simulink model "FLWSim_PoincareMap"  (R2017b)
settings: Solver=ode45  StartTime=0.0  StopTime=30  MaxStep=0.001  RelTol=1e-3
InitFcn:
  | SimInit
  | PolyRegressionFilterInit
  | CustomInit
undefined symbols (not defined in the file): dq, IC, q, sample_time
libraries: commchan3 x8, simulink x2, dspsigattribs x2
settings Model: Creator=81068  LastModifiedBy=81068
settings SFSimCC: SimUserSources=|
  | CoriolisTerm_src.c
  | GravityVector_src.c
  | InertiaMatrix_src.c
  | 
  | AMBody_LeftShin_src.c
  | AMBody_LeftThigh_src.c
  | AMBody_RightShin_src.c
  | AMBody_RightThigh_src.c
  | AMBody_Torso_src.c
  | AMworld_about_pA_src.c
  | AMWorld_LeftShin_src.c
  | AMWorld_LeftThigh_src.c
  | AMWorld_RightShin_src.c
  | AMWorld_RightThigh_src.c
  | AMWorld_Torso_src.c
  | dJb_Head_src.c
  | dJb_LeftHip_src.c
  | dJb_LeftKnee_src.c
  | dJb_LeftShin_src.c
  | dJb_LeftThigh_src.c
  | dJb_LeftToe_src.c
  | dJb_RightHip_src.c
  | dJb_RightKnee_src.c
  | dJb_RightShin_src.c
  | dJb_RightThigh_src.c
  | dJb_RightToe_src.c
  | dJb_Torso_src.c
  | dJp_COM_src.c
  | dJp_Head_src.c
  | dJp_LeftHip_src.c
  | dJp_LeftKnee_src.c
  | dJp_LeftShin_src.c
  | dJp_LeftThigh_src.c
  | dJp_LeftToe_src.c
  | dJp_RightHip_src.c
  | dJp_RightKnee_src.c
  | dJp_RightShin_src.c
  | dJp_RightThigh_src.c
  | dJp_RightToe_src.c
  | dJp_Torso_src.c
  | dJs_Head_src.c
  | dJs_LeftHip_src.c
  | dJs_LeftKnee_src.c
  | dJs_LeftShin_src.c
  | dJs_LeftThigh_src.c
  | dJs_LeftToe_src.c
  | dJs_RightHip_src.c
  | dJs_RightKnee_src.c
  | dJs_RightShin_src.c
  | dJs_RightThigh_src.c
  | dJs_RightToe_src.c
  | dJs_Torso_src.c
  | dR_Head_src.c
  | dR_LeftHip_src.c
  | dR_LeftKnee_src.c
  | dR_LeftShin_src.c
  | dR_LeftThigh_src.c
  | dR_LeftToe_src.c
  | dR_RightHip_src.c
  | dR_RightKnee_src.c
  | dR_RightShin_src.c
  | dR_RightThigh_src.c
  | dR_RightToe_src.c
  | dR_Torso_src.c
  | dT_Head_src.c
  | dT_LeftHip_src.c
  | dT_LeftKnee_src.c
  | dT_LeftShin_src.c
  | dT_LeftThigh_src.c
  | dT_LeftToe_src.c
  | dT_RightHip_src.c
  | dT_RightKnee_src.c
  | dT_RightShin_src.c
  | dT_RightThigh_src.c
  | dT_RightToe_src.c
  | dT_Torso_src.c
  | Inertia_LeftShin_src.c
  | Inertia_LeftThigh_src.c
  | Inertia_RightShin_src.c
  | Inertia_RightThigh_src.c
  | Inertia_Torso_src.c
  | Jb_Head_src.c
  | Jb_LeftHip_src.c
  | Jb_LeftKnee_src.c
  | Jb_LeftShin_src.c
  | Jb_LeftThigh_src.c
  | Jb_LeftToe_src.c
  | Jb_RightHip_src.c
  | Jb_RightKnee_src.c
  | Jb_RightShin_src.c
  | Jb_RightThigh_src.c
  | Jb_RightToe_src.c
  | Jb_Torso_src.c
  | Jdq_AMBody_LeftShin_src.c
  | Jdq_AMBody_LeftThigh_src.c
  | Jdq_AMBody_RightShin_src.c
  | Jdq_AMBody_RightThigh_src.c
  | Jdq_AMBody_Torso_src.c
  | Jdq_AMworld_about_pA_src.c
  | Jdq_AMWorld_LeftShin_src.c
  | Jdq_AMWorld_LeftThigh_src.c
  | Jdq_AMWorld_RightShin_src.c
  | Jdq_AMWorld_RightThigh_src.c
  | Jdq_AMWorld_Torso_src.c
  | Jp_COM_src.c
  | Jp_Head_src.c
  | Jp_LeftHip_src.c
  | Jp_LeftKnee_src.c
  | Jp_LeftShin_src.c
  | Jp_LeftThigh_src.c
  | Jp_LeftToe_src.c
  | Jp_RightHip_src.c
  | Jp_RightKnee_src.c
  | Jp_RightShin_src.c
  | Jp_RightThigh_src.c
  | Jp_RightToe_src.c
  | Jp_Torso_src.c
  | Jq_AMBody_LeftShin_src.c
  | Jq_AMBody_LeftThigh_src.c
  | Jq_AMBody_RightShin_src.c
  | Jq_AMBody_RightThigh_src.c
  | Jq_AMBody_Torso_src.c
  | Jq_AMworld_about_pA_src.c
  | Jq_AMWorld_LeftShin_src.c
  | Jq_AMWorld_LeftThigh_src.c
  | Jq_AMWorld_RightShin_src.c
  | Jq_AMWorld_RightThigh_src.c
  | Jq_AMWorld_Torso_src.c
  | Js_Head_src.c
  | Js_LeftHip_src.c
  | Js_LeftKnee_src.c
  | Js_LeftShin_src.c
  | Js_LeftThigh_src.c
  | Js_LeftToe_src.c
  | Js_RightHip_src.c
  | Js_RightKnee_src.c
  | Js_RightShin_src.c
  | Js_RightThigh_src.c
  | Js_RightToe_src.c
  | Js_Torso_src.c
  | p_COM_src.c
  | p_Head_src.c
  | p_LeftHip_src.c
  | p_LeftKnee_src.c
  | p_LeftShin_src.c
  | p_LeftThigh_src.c
  | p_LeftToe_src.c
  | p_RightHip_src.c
  | p_RightKnee_src.c
  | p_RightShin_src.c
  | p_RightThigh_src.c
  | p_RightToe_src.c
  | p_Torso_src.c
  | R_Head_src.c
  | R_LeftHip_src.c
  | R_LeftKnee_src.c
  | R_LeftShin_src.c
  | R_LeftThigh_src.c
  | R_LeftToe_src.c
  | R_RightHip_src.c
  | R_RightKnee_src.c
  | R_RightShin_src.c
  | R_RightThigh_src.c
  | R_RightToe_src.c
  | R_Torso_src.c
  | T_Head_src.c
  | T_LeftHip_src.c
  | T_LeftKnee_src.c
  | T_LeftShin_src.c
  | T_LeftThigh_src.c
  | T_LeftToe_src.c
  | T_RightHip_src.c
  | T_RightKnee_src.c
  | T_RightShin_src.c
  | T_RightThigh_src.c
  | T_RightToe_src.c
  | T_Torso_src.c
settings SFSimCC: SimUserIncludeDirs=|
  | .\dyn\src
  | .\kin\src
settings RTWCC: RTWUseSimCustomCode=on
settings RTWCC: CustomInclude=|
  | .\dyn\src
  | .\kin\src
settings RTWCC: CustomSource=|
  | CoriolisTerm_src.c
  | GravityVector_src.c
  | InertiaMatrix_src.c
  | 
  | AMBody_LeftShin_src.c
  | AMBody_LeftThigh_src.c
  | AMBody_RightShin_src.c
  | AMBody_RightThigh_src.c
  | AMBody_Torso_src.c
  | AMworld_about_pA_src.c
  | AMWorld_LeftShin_src.c
  | AMWorld_LeftThigh_src.c
  | AMWorld_RightShin_src.c
  | AMWorld_RightThigh_src.c
  | AMWorld_Torso_src.c
  | dJb_Head_src.c
  | dJb_LeftHip_src.c
  | dJb_LeftKnee_src.c
  | dJb_LeftShin_src.c
  | dJb_LeftThigh_src.c
  | dJb_LeftToe_src.c
  | dJb_RightHip_src.c
  | dJb_RightKnee_src.c
  | dJb_RightShin_src.c
  | dJb_RightThigh_src.c
  | dJb_RightToe_src.c
  | dJb_Torso_src.c
  | dJp_COM_src.c
  | dJp_Head_src.c
  | dJp_LeftHip_src.c
  | dJp_LeftKnee_src.c
  | dJp_LeftShin_src.c
  | dJp_LeftThigh_src.c
  | dJp_LeftToe_src.c
  | dJp_RightHip_src.c
  | dJp_RightKnee_src.c
  | dJp_RightShin_src.c
  | dJp_RightThigh_src.c
  | dJp_RightToe_src.c
  | dJp_Torso_src.c
  | dJs_Head_src.c
  | dJs_LeftHip_src.c
  | dJs_LeftKnee_src.c
  | dJs_LeftShin_src.c
  | dJs_LeftThigh_src.c
  | dJs_LeftToe_src.c
  | dJs_RightHip_src.c
  | dJs_RightKnee_src.c
  | dJs_RightShin_src.c
  | dJs_RightThigh_src.c
  | dJs_RightToe_src.c
  | dJs_Torso_src.c
  | dR_Head_src.c
  | dR_LeftHip_src.c
  | dR_LeftKnee_src.c
  | dR_LeftShin_src.c
  | dR_LeftThigh_src.c
  | dR_LeftToe_src.c
  | dR_RightHip_src.c
  | dR_RightKnee_src.c
  | dR_RightShin_src.c
  | dR_RightThigh_src.c
  | dR_RightToe_src.c
  | dR_Torso_src.c
  | dT_Head_src.c
  | dT_LeftHip_src.c
  | dT_LeftKnee_src.c
  | dT_LeftShin_src.c
  | dT_LeftThigh_src.c
  | dT_LeftToe_src.c
  | dT_RightHip_src.c
  | dT_RightKnee_src.c
  | dT_RightShin_src.c
  | dT_RightThigh_src.c
  | dT_RightToe_src.c
  | dT_Torso_src.c
  | Inertia_LeftShin_src.c
  | Inertia_LeftThigh_src.c
  | Inertia_RightShin_src.c
  | Inertia_RightThigh_src.c
  | Inertia_Torso_src.c
  | Jb_Head_src.c
  | Jb_LeftHip_src.c
  | Jb_LeftKnee_src.c
  | Jb_LeftShin_src.c
  | Jb_LeftThigh_src.c
  | Jb_LeftToe_src.c
  | Jb_RightHip_src.c
  | Jb_RightKnee_src.c
  | Jb_RightShin_src.c
  | Jb_RightThigh_src.c
  | Jb_RightToe_src.c
  | Jb_Torso_src.c
  | Jdq_AMBody_LeftShin_src.c
  | Jdq_AMBody_LeftThigh_src.c
  | Jdq_AMBody_RightShin_src.c
  | Jdq_AMBody_RightThigh_src.c
  | Jdq_AMBody_Torso_src.c
  | Jdq_AMworld_about_pA_src.c
  | Jdq_AMWorld_LeftShin_src.c
  | Jdq_AMWorld_LeftThigh_src.c
  | Jdq_AMWorld_RightShin_src.c
  | Jdq_AMWorld_RightThigh_src.c
  | Jdq_AMWorld_Torso_src.c
  | Jp_COM_src.c
  | Jp_Head_src.c
  | Jp_LeftHip_src.c
  | Jp_LeftKnee_src.c
  | Jp_LeftShin_src.c
  | Jp_LeftThigh_src.c
  | Jp_LeftToe_src.c
  | Jp_RightHip_src.c
  | Jp_RightKnee_src.c
  | Jp_RightShin_src.c
  | Jp_RightThigh_src.c
  | Jp_RightToe_src.c
  | Jp_Torso_src.c
  | Jq_AMBody_LeftShin_src.c
  | Jq_AMBody_LeftThigh_src.c
  | Jq_AMBody_RightShin_src.c
  | Jq_AMBody_RightThigh_src.c
  | Jq_AMBody_Torso_src.c
  | Jq_AMworld_about_pA_src.c
  | Jq_AMWorld_LeftShin_src.c
  | Jq_AMWorld_LeftThigh_src.c
  | Jq_AMWorld_RightShin_src.c
  | Jq_AMWorld_RightThigh_src.c
  | Jq_AMWorld_Torso_src.c
  | Js_Head_src.c
  | Js_LeftHip_src.c
  | Js_LeftKnee_src.c
  | Js_LeftShin_src.c
  | Js_LeftThigh_src.c
  | Js_LeftToe_src.c
  | Js_RightHip_src.c
  | Js_RightKnee_src.c
  | Js_RightShin_src.c
  | Js_RightThigh_src.c
  | Js_RightToe_src.c
  | Js_Torso_src.c
  | p_COM_src.c
  | p_Head_src.c
  | p_LeftHip_src.c
  | p_LeftKnee_src.c
  | p_LeftShin_src.c
  | p_LeftThigh_src.c
  | p_LeftToe_src.c
  | p_RightHip_src.c
  | p_RightKnee_src.c
  | p_RightShin_src.c
  | p_RightThigh_src.c
  | p_RightToe_src.c
  | p_Torso_src.c
  | R_Head_src.c
  | R_LeftHip_src.c
  | R_LeftKnee_src.c
  | R_LeftShin_src.c
  | R_LeftThigh_src.c
  | R_LeftToe_src.c
  | R_RightHip_src.c
  | R_RightKnee_src.c
  | R_RightShin_src.c
  | R_RightThigh_src.c
  | R_RightToe_src.c
  | R_Torso_src.c
  | T_Head_src.c
  | T_LeftHip_src.c
  | T_LeftKnee_src.c
  | T_LeftShin_src.c
  | T_LeftThigh_src.c
  | T_LeftToe_src.c
  | T_RightHip_src.c
  | T_RightKnee_src.c
  | T_RightShin_src.c
  | T_RightThigh_src.c
  | T_RightToe_src.c
  | T_Torso_src.c
settings CodeAppCC: StateflowObjectComments=on

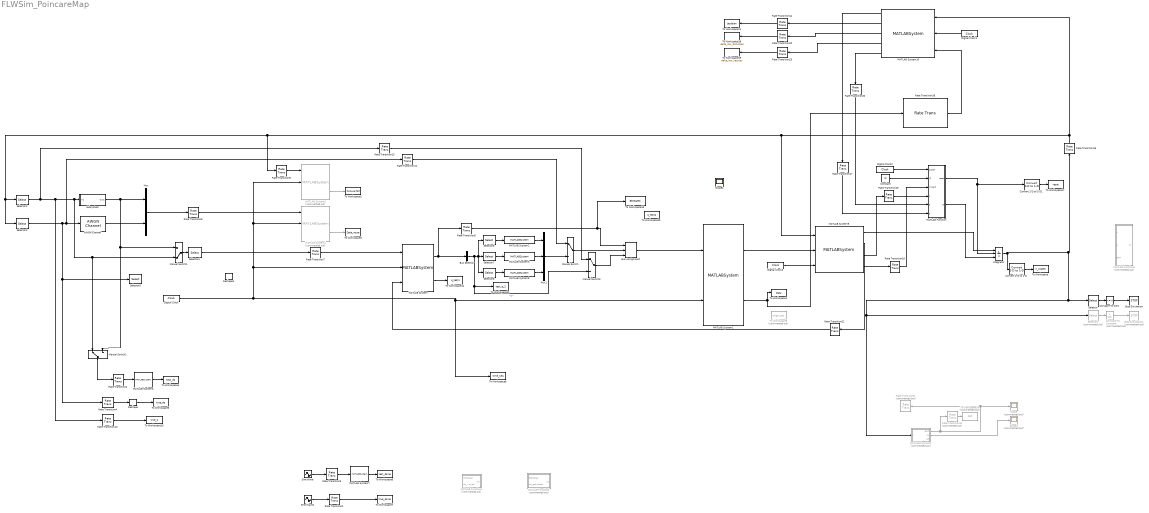
== system FLWSim_PoincareMap ==
  AWGN Channel : commchan3/AWGN Channel  InputProcessing=Columns as channels (frame based)  seed=4  noiseMode=Variance from mask  EbNodB=10  EsNodB=10  SNRdB=10  bitsPerSym=1  Ps=1  Tsym=1  variance=cov_dq_estimated
  Bus Assignment : BusAssignment  AssignedSignals=dq,q
  Bus Selector : BusSelector  OutputSignals=q
  Compare To Constant : simulink/Logic and Bit Operations/Compare To Constant  Commented=on  relop=>  const=100  OutDataTypeStr=boolean
  Compare To Zero : simulink/Logic and Bit Operations/Compare To Zero  relop=<=  OutDataTypeStr=boolean
  Constant : Constant  Value=IC
  Convert 2-D to 1-D : dspsigattribs/Convert 2-D to 1-D
      settings: SourceProductName=DSP System Toolbox  SourceProductBaseCode=DS
  Convert 2-D to 1-D1 : dspsigattribs/Convert 2-D to 1-D
      settings: SourceProductName=DSP System Toolbox  SourceProductBaseCode=DS
  Digital Clock{,1..3} (4 alike) : DigitalClock  SampleTime=sample_time
  Integrator : Integrator  ExternalReset=level hold  InitialConditionSource=external  InitialCondition=IC
  MATLAB Function : MATLAB Function  TreatAsAtomicUnit=on
  MATLAB Function1 : MATLAB Function  Commented=on  TreatAsAtomicUnit=on
  MATLAB Function4 : MATLAB Function  Commented=on  TreatAsAtomicUnit=on
  MATLAB Function5 : MATLAB Function  Commented=on  TreatAsAtomicUnit=on
  MATLAB Function6 : MATLAB Function  Commented=on  TreatAsAtomicUnit=on
  MATLAB System : MATLABSystem  System=StateEstimator_1  T=0.3  SimulateUsing=Interpreted execution
      mask Type: StateEstimator_1
      mask Display:
      | disp('StateEstimator_1');
      | port_label('input',1,'q_measured');
      | port_label('input',2,'t');
      | port_label('input',3,'GRF');
      | port_label('output',1,'EstStates');
      | port_label('output',2,'q');
  MATLAB System1 : MATLABSystem  System=FLW_Controller_Poincare  cov_q_measured=cov_q_measured  cov_dq_estimated=cov_dq_estimated  T_sample=sample_time  T=0.3  RegressFilterHistoryLength=history_length  fp_ratio=fp_ratio  SimulateUsing=Code generation
      mask Type: FLW_Controller_Poincare
      mask Display:
      | disp('FLW_Controller_Poincare');
      | port_label('input',1,'EstStates');
      | port_label('input',2,'t');
      | port_label('output',1,'u');
      | port_label('output',2,'Data');
  MATLAB System10 : MATLABSystem  System=Poincare_test  poincare_delta=poincare_delta  SimulateUsing=Code generation
      mask Type: Poincare_test
      mask Display:
      | disp('Poincare_test');
      | port_label('input',1,'x');
      | port_label('input',2,'t_total');
      | port_label('input',3,'Data');
      | port_label('output',1,'x_out');
      | port_label('output',2,'Jacobian');
      | port_label('output',3,'delta_low_disturbed');
      | port_label('output',4,'delta_low_recover');
      | port_label('output',5,'add_disturb');
  MATLAB System2 : MATLABSystem  System=PolyRegressionFilter  sample_time=sample_time  history_length=history_length  dop=dop  signal_dim=2  delay=RegressionDelay  SimulateUsing=Code generation
      mask Type: PolyRegressionFilter
      mask Display:
      | disp('PolyRegressionFilter');
      | port_label('input',1,'q');
      | port_label('output',1,'dq');
  MATLAB System3 : MATLABSystem  System=PolyRegressionFilter  sample_time=sample_time  history_length=history_length  dop=dop  signal_dim=1  delay=RegressionDelay  SimulateUsing=Code generation
      mask Type: PolyRegressionFilter
      mask Display:
      | disp('PolyRegressionFilter');
      | port_label('input',1,'q');
      | port_label('output',1,'dq');
  MATLAB System4 : MATLABSystem  Commented=on  System=FLW_Controller_3  cov_q=cov_q_measured  cov_dq=cov_dq_estimated  T_sample=sample_time  SimulateUsing=Code generation
      mask Type: FLW_Controller_3
      mask Display:
      | disp('FLW_Controller_3');
      | port_label('input',1,'x');
      | port_label('input',2,'t');
      | port_label('input',3,'GRF');
      | port_label('output',1,'u');
      | port_label('output',2,'Data');
  MATLAB System5 : MATLABSystem  Commented=on  System=FLW_Controller_3  cov_q=cov_q_measured  cov_dq=cov_dq_estimated  T_sample=sample_time  SimulateUsing=Code generation
      mask Type: FLW_Controller_3
      mask Display:
      | disp('FLW_Controller_3');
      | port_label('input',1,'x');
      | port_label('input',2,'t');
      | port_label('input',3,'GRF');
      | port_label('output',1,'u');
      | port_label('output',2,'Data');
  MATLAB System6 : MATLABSystem  System=PolyRegressionFilter  sample_time=sample_time  history_length=history_length  dop=dop  signal_dim=7  delay=RegressionDelay  SimulateUsing=Code generation
      mask Type: PolyRegressionFilter
      mask Display:
      | disp('PolyRegressionFilter');
      | port_label('input',1,'q');
      | port_label('output',1,'dq');
  MATLAB System7 : MATLABSystem  System=PolyRegressionFilter  sample_time=sample_time  history_length=history_length  dop=dop  signal_dim=1  delay=20  SimulateUsing=Code generation
      mask Type: PolyRegressionFilter
      mask Display:
      | disp('PolyRegressionFilter');
      | port_label('input',1,'q');
      | port_label('output',1,'dq');
  MATLAB System8 : MATLABSystem  System=PolyRegressionFilter  sample_time=sample_time  history_length=history_length  dop=dop  signal_dim=4  delay=RegressionDelay  SimulateUsing=Code generation
      mask Type: PolyRegressionFilter
      mask Display:
      | disp('PolyRegressionFilter');
      | port_label('input',1,'q');
      | port_label('output',1,'dq');
  MATLAB System9 : MATLABSystem  System=EOM_Rigid_Ground  IC=IC  SimulateUsing=Code generation
      mask Type: EOM_Rigid_Ground
      mask Display:
      | disp('EOM_Rigid_Ground');
      | port_label('input',1,'x');
      | port_label('input',2,'u');
      | port_label('input',3,'t_total');
      | port_label('output',1,'dx');
      | port_label('output',2,'GRF');
      | port_label('output',3,'x_reset');
      | port_label('output',4,'impact');
  Manual Switch : ManualSwitch
  Manual Switch1 : ManualSwitch  CurrentSetting=0
  Manual Switch2 : ManualSwitch
  Manual Switch3 : ManualSwitch
  Mux : Mux  Inputs=2
  Mux1 : Mux  Inputs=3
  Rate Transition{1..8,10..11,13..15,22..23} (15 alike) : RateTransition  OutPortSampleTime=sample_time
  Rate Transition12 : RateTransition  Commented=on  OutPortSampleTime=sample_time
  Rate Transition{16..21} (6 alike) : RateTransition  OutPortSampleTimeOpt=Inherit
  Rate Transition9 : RateTransition  Commented=on  OutPortSampleTime=sample_time
  Reshape : Reshape  OutputDimensionality=Column vector (2-D)
  Reshape1 : Reshape  OutputDimensionality=Column vector (2-D)
  Scope : Scope  Commented=on
  Scope1 : Scope  Commented=on
  Scope2 : Scope
  Selector : Selector  InputPortWidth=14  IndexOptions=Index vector (dialog)  Indices=[2]  OutputSizes=1
  Selector1 : Selector  Commented=on  InputPortWidth=14  IndexOptions=Index vector (dialog)  Indices=[8]  OutputSizes=1
  Selector2 : Selector  InputPortWidth=14  IndexOptions=Index vector (dialog)  Indices=[1:7]  OutputSizes=1
  Selector3 : Selector  InputPortWidth=14  IndexOptions=Index vector (dialog)  Indices=[8:14]  OutputSizes=1
  Selector4 : Selector  InputPortWidth=7  IndexOptions=Index vector (dialog)  Indices=[3:7]  OutputSizes=1
  Selector5 : Selector  InputPortWidth=7  IndexOptions=Index vector (dialog)  Indices=[3:7]  OutputSizes=1
  Selector6 : Selector  InputPortWidth=7  IndexOptions=Index vector (dialog)  Indices=[1:2]  OutputSizes=1
  Selector7 : Selector  InputPortWidth=7  IndexOptions=Index vector (dialog)  Indices=[3]  OutputSizes=1
  Selector8 : Selector  InputPortWidth=7  IndexOptions=Index vector (dialog)  Indices=[4:7]  OutputSizes=1
  Sine Wave : Sin  Frequency=10  SampleTime=0
  Sine Wave1 : Sin  Amplitude=10  Frequency=10  Phase=pi/2  SampleTime=0
  Stop Simulation : Stop
  Stop Simulation1 : Stop  Commented=on
  Subsystem : Subsystem
  To Workspace : ToWorkspace  VariableName=X_states  SampleTime=-1
  To Workspace1 : ToWorkspace  VariableName=Data  SaveFormat=Timeseries  SampleTime=-1
  To Workspace10 : ToWorkspace  VariableName=true_q  SaveFormat=Timeseries  SampleTime=-1
  To Workspace11 : ToWorkspace  VariableName=Jacobian  SampleTime=-1
  To Workspace12 : ToWorkspace  VariableName=test_q_2  SaveFormat=Timeseries  SampleTime=-1
  To Workspace13 : ToWorkspace  VariableName=EstStates  SaveFormat=Timeseries  SampleTime=-1
  To Workspace14 : ToWorkspace  VariableName=q_test1  SaveFormat=Timeseries  SampleTime=-1
  To Workspace15 : ToWorkspace  VariableName=q_test2  SaveFormat=Timeseries  SampleTime=-1
  To Workspace16 : ToWorkspace  Commented=on  VariableName=GRF  SaveFormat=Timeseries  SampleTime=-1
  To Workspace17 : ToWorkspace  VariableName=reset  SampleTime=-1
  To Workspace18 : ToWorkspace  VariableName=delta_low_disturbed  SampleTime=-1
  To Workspace19 : ToWorkspace  VariableName=delta_low_recover  SampleTime=-1
  To Workspace2 : ToWorkspace  VariableName=Data_perfect  SaveFormat=Timeseries  SampleTime=-1
  To Workspace3 : ToWorkspace  VariableName=Data_noise  SaveFormat=Timeseries  SampleTime=-1
  To Workspace4 : ToWorkspace  VariableName=test_dq  SaveFormat=Timeseries  SampleTime=-1
  To Workspace5 : ToWorkspace  VariableName=true_dq  SaveFormat=Timeseries  SampleTime=-1
  To Workspace6 : ToWorkspace  VariableName=test_dsine  SaveFormat=Timeseries  SampleTime=-1
  To Workspace7 : ToWorkspace  VariableName=true_dsine  SaveFormat=Timeseries  SampleTime=-1
  To Workspace8 : ToWorkspace  VariableName=time_seq  SampleTime=-1
      settings: Save2DSignal=2-D array (concatenate along first dimension)
  To Workspace9 : ToWorkspace  Commented=on  VariableName=origin_pos  SaveFormat=Timeseries  SampleTime=-1
  wires:
  MATLAB Function1/2(pL) -> Scope1/1
  Compare To Zero/1 -> Stop Simulation/1
  Selector/1 -> Compare To Zero/1
  Digital Clock/1 -> MATLAB System/2, MATLAB System5/2, MATLAB System4/2, To Workspace8/1, MATLAB System1/2
  Selector1/1 -> Compare To Constant/1
  Compare To Constant/1 -> Stop Simulation1/1
  MATLAB System5/2 -> To Workspace2/1
  MATLAB System4/2 -> To Workspace3/1
  Mux/1 -> Rate Transition8/1
  AWGN Channel/1 -> Mux/2
  Selector3/1 -> Rate Transition11/1, AWGN Channel/1, Selector5/1, Rate Transition4/1
  Selector2/1 -> Rate Transition13/1, Subsystem/1(In1), Manual Switch2/1, Manual Switch1/2, Rate Transition10/1
  Subsystem/1(Out1) -> Manual Switch2/2, Manual Switch1/1, Mux/1
  Rate Transition2/1 -> MATLAB System6/1
  MATLAB System6/1 -> To Workspace4/1
  Sine Wave/1 -> Rate Transition3/1
  Rate Transition3/1 -> MATLAB System7/1
  MATLAB System7/1 -> To Workspace6/1
  Sine Wave1/1 -> Rate Transition1/1
  Rate Transition4/1 -> Reshape/1
  Reshape/1 -> To Workspace5/1
  Selector4/1 -> Rate Transition7/1
  Manual Switch1/1 -> Selector4/1
  Rate Transition6/1 -> MATLAB System5/1
  Rate Transition1/1 -> To Workspace7/1
  Rate Transition8/1 -> MATLAB System4/1
  Manual Switch2/1 -> Rate Transition2/1
  MATLAB System2/1 -> Mux1/1
  Selector6/1 -> MATLAB System2/1
  Selector8/1 -> MATLAB System8/1
  Bus Selector/1 -> Manual Switch3/2, To Workspace12/1, Selector8/1, Selector7/1, Selector6/1  "<q>"
  MATLAB System/1 -> Rate Transition5/1, Bus Selector/1
  Rate Transition7/1 -> MATLAB System/1
  Selector7/1 -> MATLAB System3/1
  MATLAB System8/1 -> Mux1/3
  MATLAB System3/1 -> Mux1/2
  Mux1/1 -> Manual Switch/2
  Rate Transition5/1 -> To Workspace13/1, Bus Assignment/1
  Manual Switch/1 -> Bus Assignment/2
  MATLAB Function1/1(GRF) -> Rate Transition12/1, Rate Transition9/1, Scope/1
  Bus Assignment/1 -> MATLAB System1/1
  MATLAB System/2 -> To Workspace14/1
  ? -> MATLAB Function4/1(EstStates)
  ? -> MATLAB Function4/2(dq_measured)
  Rate Transition11/1 -> Manual Switch/1
  Rate Transition10/1 -> To Workspace10/1
  Rate Transition12/1 -> To Workspace16/1
  Manual Switch3/1 -> Bus Assignment/3
  Rate Transition13/1 -> Manual Switch3/1
  Digital Clock1/1 -> MATLAB System10/2
  MATLAB System10/2 -> Rate Transition14/1
  Rate Transition14/1 -> To Workspace11/1
  Integrator/1 -> MATLAB Function1/1(x), Selector1/1, Selector/1, Rate Transition15/1, Convert 2-D to 1-D/1
  MATLAB System1/2 -> Rate Transition16/1, To Workspace1/1
  Rate Transition16/1 -> MATLAB System10/3
  Convert 2-D to 1-D/1 -> To Workspace/1
  MATLAB System9/1 -> Integrator/1
  MATLAB System1/1 -> MATLAB System9/2
  Digital Clock3/1 -> MATLAB System9/3
  Convert 2-D to 1-D1/1 -> To Workspace17/1
  Constant/1 -> MATLAB Function/2(IC)
  Digital Clock2/1 -> MATLAB Function/1(t_total)
  MATLAB Function/1(reset) -> Integrator/2, Convert 2-D to 1-D1/1
  MATLAB Function/2(x0) -> Integrator/3
  Rate Transition18/1 -> MATLAB Function/3(impact)
  Rate Transition19/1 -> MATLAB Function/4(x_impact_reset)
  Rate Transition15/1 -> MATLAB System9/1, Rate Transition6/1, Selector2/1, Selector3/1, MATLAB System10/1
  MATLAB System10/1 -> Rate Transition17/1
  Rate Transition17/1 -> MATLAB Function/6(x_poincare_reset)
  Rate Transition20/1 -> MATLAB Function/5(poincare_disturb)
  MATLAB System9/4 -> Rate Transition18/1
  MATLAB System9/3 -> Rate Transition19/1
  MATLAB System9/2 -> Rate Transition21/1
  Rate Transition21/1 -> MATLAB System/3
  MATLAB System10/5 -> Rate Transition20/1
  MATLAB System10/3 -> Rate Transition22/1
  Rate Transition22/1 -> To Workspace18/1
  Rate Transition23/1 -> To Workspace19/1
  MATLAB System10/4 -> Rate Transition23/1

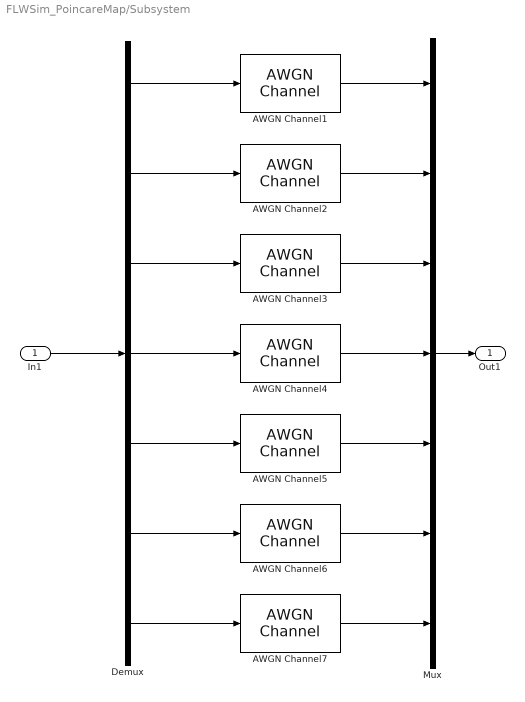
== system FLWSim_PoincareMap/Subsystem ==
  In1 : Inport
  AWGN Channel1 : commchan3/AWGN Channel  InputProcessing=Columns as channels (frame based)  seed=1  noiseMode=Variance from mask  EbNodB=10  EsNodB=10  SNRdB=10  bitsPerSym=1  Ps=1  Tsym=1  variance=cov_q_measured
  AWGN Channel2 : commchan3/AWGN Channel  InputProcessing=Columns as channels (frame based)  seed=2  noiseMode=Variance from mask  EbNodB=10  EsNodB=10  SNRdB=10  bitsPerSym=1  Ps=1  Tsym=1  variance=cov_q_measured
  AWGN Channel3 : commchan3/AWGN Channel  InputProcessing=Columns as channels (frame based)  seed=3  noiseMode=Variance from mask  EbNodB=10  EsNodB=10  SNRdB=10  bitsPerSym=1  Ps=1  Tsym=1  variance=cov_q_measured
  AWGN Channel4 : commchan3/AWGN Channel  InputProcessing=Columns as channels (frame based)  seed=4  noiseMode=Variance from mask  EbNodB=10  EsNodB=10  SNRdB=10  bitsPerSym=1  Ps=1  Tsym=1  variance=cov_q_measured
  AWGN Channel5 : commchan3/AWGN Channel  InputProcessing=Columns as channels (frame based)  seed=5  noiseMode=Variance from mask  EbNodB=10  EsNodB=10  SNRdB=10  bitsPerSym=1  Ps=1  Tsym=1  variance=cov_q_measured
  AWGN Channel6 : commchan3/AWGN Channel  InputProcessing=Columns as channels (frame based)  seed=6  noiseMode=Variance from mask  EbNodB=10  EsNodB=10  SNRdB=10  bitsPerSym=1  Ps=1  Tsym=1  variance=cov_q_measured
  AWGN Channel7 : commchan3/AWGN Channel  InputProcessing=Columns as channels (frame based)  seed=7  noiseMode=Variance from mask  EbNodB=10  EsNodB=10  SNRdB=10  bitsPerSym=1  Ps=1  Tsym=1  variance=cov_q_measured
  Demux : Demux  Outputs=7
  Mux : Mux  Inputs=7
  Out1 : Outport
  wires:
  In1/1 -> Demux/1
  Demux/1 -> AWGN Channel1/1
  Demux/2 -> AWGN Channel2/1
  Demux/3 -> AWGN Channel3/1
  Demux/4 -> AWGN Channel4/1
  Demux/5 -> AWGN Channel5/1
  Demux/6 -> AWGN Channel6/1
  Demux/7 -> AWGN Channel7/1
  AWGN Channel1/1 -> Mux/1
  AWGN Channel2/1 -> Mux/2
  AWGN Channel3/1 -> Mux/3
  AWGN Channel4/1 -> Mux/4
  AWGN Channel5/1 -> Mux/5
  AWGN Channel6/1 -> Mux/6
  AWGN Channel7/1 -> Mux/7
  Mux/1 -> Out1/1

== matlab function FLWSim_PoincareMap/MATLAB Function1 ==
  data: x input; GRF output; pL output; pR output
function [GRF,pL,pR] = fcn(x)
stiffness_v = 60000;
damping_v = 1000;
damping_h = 10000;
FC = 10; % Friction Cone
q = x(1:7);
dq = x(8:14);
GRF= zeros(6,1);

pL = p_LeftToe(q);
pR = p_RightToe(q);
vL = Jp_LeftToe(q)*dq;
vR = Jp_RightToe(q)*dq;



if pL(3)<0
    GRF_Lx = -damping_h*vL(1);
    GRF_Lz = -stiffness_v*pL(3)-damping_v*vL(3);
    GRF(1) = GRF_Lx;
    GRF(3) = GRF_Lz;
end

if pR(3)<0
    GRF_Rx = -damping_h*vR(1);
    GRF_Rz = -stiffness_v*pR(3)-damping_v*vR(3);
    GRF(4) = GRF_Rx;
    GRF(6) = GRF_Rz;
end

GRF(3) = max([0,GRF(3)]);
GRF(6) = max([0,GRF(6)]);

GRF(1) = median([GRF(1), FC*GRF(3), - FC*GRF(3)]);
GRF(4) = median([GRF(4), FC*GRF(6), - FC*GRF(6)]);
end

== matlab function FLWSim_PoincareMap/MATLAB Function ==
  data: reset output; t_total input; x0 output; IC input; impact input; x_impact_reset input; poincare_disturb input; x_poincare_reset input
function [reset,x0] = set_IC(t_total, IC, impact,x_impact_reset, poincare_disturb, x_poincare_reset)
% function [reset,x0] = set_IC(t_total, IC, impact,x_impact_reset)
x0 = zeros(14,1);
initialize = t_total<0.001;
reset = initialize||impact||poincare_disturb;
% reset = initialize||impact;
if impact
    x0 = x_impact_reset;
end

if initialize
    x0 = IC;
end

if poincare_disturb
    x0 = x_poincare_reset;
end

== matlab function FLWSim_PoincareMap/MATLAB Function4 ==
  data: EstStates input; dq output; dq_measured input
function dq = fcn(EstStates,dq_measured)
q = EstStates.q;
q_pre = [0;0;q(3:7)];
dq_pre = [0;0;dq_measured(3:7)];
Jp_LT_pre = Jp_LeftToe(q_pre);
Jp_RT_pre = Jp_RightToe(q_pre);
rv_Hip2LT = -Jp_LT_pre*dq_pre;
rv_Hip2RT = -Jp_RT_pre*dq_pre;
if EstStates.stanceLeg == -1
    origin_vel = rv_Hip2LT;
else
    origin_vel = rv_Hip2RT;
end
dq = [origin_vel([1,3]); dq_pre([3:7])];

== matlab function FLWSim_PoincareMap/MATLAB Function5 ==
  data: EstStates input; dq output; dq_estimated input
function dq = fcn(EstStates,dq_estimated)
q = EstStates.q;
q_pre = [0;0;q(3:7)];
dq_pre = [0;0;dq_estimated(3:7)];
Jp_LT_pre = Jp_LeftToe(q_pre);
Jp_RT_pre = Jp_RightToe(q_pre);
rv_Hip2LT = -Jp_LT_pre*dq_pre;
rv_Hip2RT = -Jp_RT_pre*dq_pre;
if EstStates.stanceLeg == -1
    origin_vel = rv_Hip2LT;
else
    origin_vel = rv_Hip2RT;
end
dq = [origin_vel([1,3]); dq_pre([3:7])];

== matlab function FLWSim_PoincareMap/MATLAB Function6 ==
  data: x input; u input; dx output; GRF input
function dx = ContinuousModel(x,u,GRF)
dx = zeros(size(x));
q = x(1:7);
dq = x(8:end);

M = InertiaMatrix(q);
C = CoriolisTerm(q,dq);
G = GravityVector(q);
B = [zeros(3,4);eye(4)];

JgL = Jp_LeftToe(q);
JgR = Jp_RightToe(q);
Jg = [JgL;JgR];

ddq = M^-1*(-C-G+B*u+Jg'*GRF);

dx = [dq;ddq];

end
